simulink model "CryoDet12Chan"  (R2016b)
settings: Solver=ode45  StartTime=0.0  StopTime=10e-4  MaxStep=1e-9  RelTol=1e-3
values from neighbouring files (symbols this model uses):
  Fclk = Fadc    (= 307200000)    [setupCryoFPGAxray.m]
  freqBusAddrBits = 4    [setupCryoFPGAxray.m]
  noise = exp(2i*pi*rand(1, noiseLen))    [setupCryoFPGAxray.m]
  noiseLen = 128    [setupCryoFPGAxray.m]
  noiseSteps = 32    [setupCryoFPGAxray.m]
  Tclk = 1/Fclk    (= 3.25520833333e-09)    [setupCryoFPGAxray.m]
undefined symbols (not defined in the file or in its folder): AXI4, Lite, notch, notch2, notch3, notch4, xlipgetpartsetting
libraries: xbsIndex_r4 x1191
(part 2 of 8)

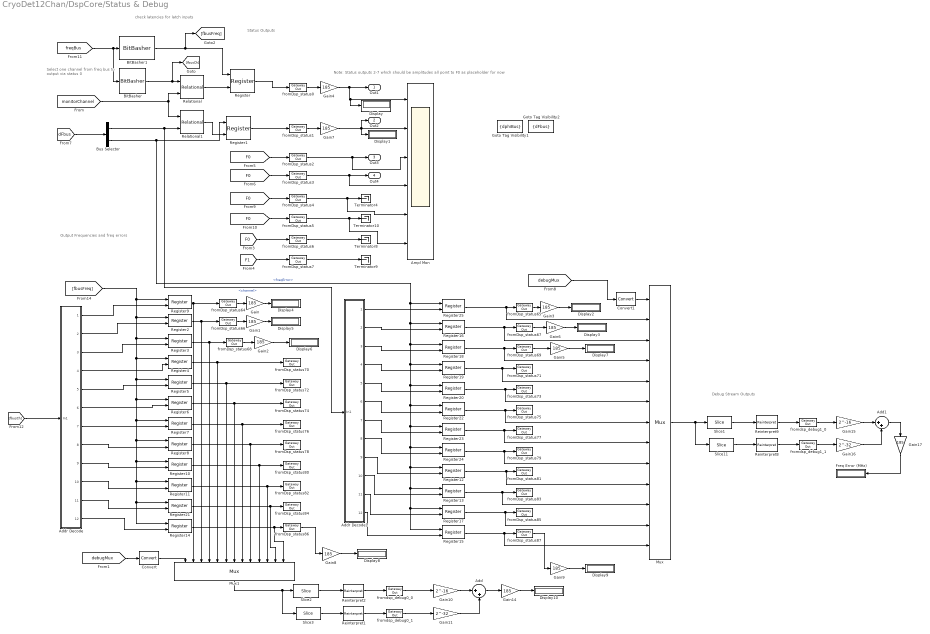
== system CryoDet12Chan/DspCore/Status & Debug ==
  note: Output Frequencies and freq errors
  note: check latencies for latch inputs
  note: Select one channel from freq bus to output via status 0
  note: Note: Status outputs 2-7 which should be amplitudes all point to F0 as placeholder for now
  note: Status Outputs
  note: Debug Stream Outputs
  Add : Sum  Inputs=|++
  Add1 : Sum  Inputs=|++
  Addr Decode : Subsystem
  Addr Decode1 : Subsystem
  Ampl Mon : Scope  NumInputPorts=6
  BitBasher : xbsIndex_r4/BitBasher  bitexpr=a={b[27:24]}  display_expr=on  sr_1=a  arith_type1=Unsigned  bin_pt1=0  sr_2=2  arith_type2=Unsigned  bin_pt2=0  sr_3=3  arith_type3=Unsigned  bin_pt3=0  sr_4=4  arith_type4=Unsigned  bin_pt4=0  dbl_ovrd=off  block_type=bitbasher
  BitBasher1 : xbsIndex_r4/BitBasher  bitexpr=a={b[23:0]}  display_expr=on  sr_1=a  arith_type1=Unsigned  bin_pt1=24  sr_2=2  arith_type2=Unsigned  bin_pt2=0  sr_3=3  arith_type3=Unsigned  bin_pt3=0  sr_4=4  arith_type4=Unsigned  bin_pt4=0  dbl_ovrd=off  block_type=bitbasher
  Bus Selector : BusSelector  OutputSignals=channel,freqError
  Convert : xbsIndex_r4/Convert  gui_display_data_type=Fixed-point  arith_type=Unsigned  n_bits=4  bin_pt=0  float_type=Single  exp_bits=8  fraction_bits=24  quantization=Truncate  overflow=Wrap  en=off  latency=1  pipeline=off  dbl_ovrd=off  block_type=convert
  Convert1 : xbsIndex_r4/Convert  gui_display_data_type=Fixed-point  arith_type=Unsigned  n_bits=4  bin_pt=0  float_type=Single  exp_bits=8  fraction_bits=24  quantization=Truncate  overflow=Wrap  en=off  latency=1  pipeline=off  dbl_ovrd=off  block_type=convert
  Display{,1..10} (11 alike) : Display
      settings: Decimation=144
  Freq Error (MHz) : Display
      settings: Decimation=144
  Gain{,1..9,14,17} (12 alike) : Gain  Gain=185
  Gain10 : Gain  Gain=2^-16
  Gain11 : Gain  Gain=2^-32
  Gain15 : Gain  Gain=2^-16
  Gain16 : Gain  Gain=2^-32
  Goto Tag Visibility1 : GotoTagVisibility  GotoTag=dphiBus
  Goto Tag Visibility2 : GotoTagVisibility  GotoTag=dFbus
  Mux : xbsIndex_r4/Mux  inputs=12  en=off  latency=0  precision=Full  arith_type=Unsigned  n_bits=16  bin_pt=14  quantization=Truncate  overflow=Wrap  dbl_ovrd=off  block_type=mux
  Mux1 : xbsIndex_r4/Mux  inputs=12  en=off  latency=0  precision=Full  arith_type=Unsigned  n_bits=16  bin_pt=14  quantization=Truncate  overflow=Wrap  dbl_ovrd=off  block_type=mux
  Register{,1..25} (26 alike) : xbsIndex_r4/Register  init=0  rst=off  en=on  dbl_ovrd=off  block_type=register
  Reinterpret{1..2,8..9} (4 alike) : xbsIndex_r4/Reinterpret  force_arith_type=on  arith_type=Unsigned  force_bin_pt=off  bin_pt=15  block_type=reinterpret
  Relational : xbsIndex_r4/Relational  mode=a=b  op_type=Bool  en=off  latency=0  dbl_ovrd=off  block_type=relational
  Relational1 : xbsIndex_r4/Relational  mode=a=b  op_type=Bool  en=off  latency=0  dbl_ovrd=off  block_type=relational
  Slice1 : xbsIndex_r4/Slice  nbits=16  boolean_output=off  mode=Upper Bit Location + Width  bit1=0  base1=MSB of Input  bit0=0  base0=LSB of Input  dbl_ovrd=off  block_type=slice
  Slice11 : xbsIndex_r4/Slice  nbits=16  boolean_output=off  mode=Lower Bit Location + Width  bit1=0  base1=MSB of Input  bit0=0  base0=LSB of Input  dbl_ovrd=off  block_type=slice
  Slice2 : xbsIndex_r4/Slice  nbits=16  boolean_output=off  mode=Upper Bit Location + Width  bit1=0  base1=MSB of Input  bit0=0  base0=LSB of Input  dbl_ovrd=off  block_type=slice
  Slice3 : xbsIndex_r4/Slice  nbits=16  boolean_output=off  mode=Lower Bit Location + Width  bit1=0  base1=MSB of Input  bit0=0  base0=LSB of Input  dbl_ovrd=off  block_type=slice
  Terminator{4,8..10} (4 alike) : Terminator
  fromDsp_status0 : xbsIndex_r4/Gateway Out  inherit_from_input=on  hdl_port=on  rows=1  columns=1  UseAsDAC=off  DACChannel='1'  interface=AXI4-Lite  automatic_assignment=off  address_offset=hex2dec('00')  intf_name=''  intf_description=''  timing_constraint=None  locs_specified=off  LOCs={}  io_standard={}  block_type=gatewayout
  fromDsp_status1 : xbsIndex_r4/Gateway Out  inherit_from_input=on  hdl_port=on  rows=1  columns=1  UseAsDAC=off  DACChannel='1'  interface=AXI4-Lite  automatic_assignment=off  address_offset=hex2dec('04')  intf_name=''  intf_description=''  timing_constraint=None  locs_specified=off  LOCs={}  io_standard={}  block_type=gatewayout
  fromDsp_status2 : xbsIndex_r4/Gateway Out  inherit_from_input=on  hdl_port=on  rows=1  columns=1  UseAsDAC=off  DACChannel='1'  interface=AXI4-Lite  automatic_assignment=off  address_offset=hex2dec('08')  intf_name=''  intf_description=''  timing_constraint=None  locs_specified=off  LOCs={}  io_standard={}  block_type=gatewayout
  fromDsp_status3 : xbsIndex_r4/Gateway Out  inherit_from_input=on  hdl_port=on  rows=1  columns=1  UseAsDAC=off  DACChannel='1'  interface=AXI4-Lite  automatic_assignment=off  address_offset=hex2dec('0C')  intf_name=''  intf_description=''  timing_constraint=None  locs_specified=off  LOCs={}  io_standard={}  block_type=gatewayout
  fromDsp_status4 : xbsIndex_r4/Gateway Out  inherit_from_input=on  hdl_port=on  rows=1  columns=1  UseAsDAC=off  DACChannel='1'  interface=AXI4-Lite  automatic_assignment=off  address_offset=hex2dec('10')  intf_name=''  intf_description=''  timing_constraint=None  locs_specified=off  LOCs={}  io_standard={}  block_type=gatewayout
  fromDsp_status5 : xbsIndex_r4/Gateway Out  inherit_from_input=on  hdl_port=on  rows=1  columns=1  UseAsDAC=off  DACChannel='1'  interface=AXI4-Lite  automatic_assignment=off  address_offset=hex2dec('14')  intf_name=''  intf_description=''  timing_constraint=None  locs_specified=off  LOCs={}  io_standard={}  block_type=gatewayout
  fromDsp_status6 : xbsIndex_r4/Gateway Out  inherit_from_input=on  hdl_port=on  rows=1  columns=1  UseAsDAC=off  DACChannel='1'  interface=AXI4-Lite  automatic_assignment=off  address_offset=hex2dec('18')  intf_name=''  intf_description=''  timing_constraint=None  locs_specified=off  LOCs={}  io_standard={}  block_type=gatewayout
  fromDsp_status64 : xbsIndex_r4/Gateway Out  inherit_from_input=on  hdl_port=on  rows=1  columns=1  UseAsDAC=off  DACChannel='1'  interface=AXI4-Lite  automatic_assignment=off  address_offset=hex2dec('100')  intf_name=''  intf_description=''  timing_constraint=None  locs_specified=off  LOCs={}  io_standard={}  block_type=gatewayout
  fromDsp_status65 : xbsIndex_r4/Gateway Out  inherit_from_input=on  hdl_port=on  rows=1  columns=1  UseAsDAC=off  DACChannel='1'  interface=AXI4-Lite  automatic_assignment=off  address_offset=hex2dec('104')  intf_name=''  intf_description=''  timing_constraint=None  locs_specified=off  LOCs={}  io_standard={}  block_type=gatewayout
  fromDsp_status66 : xbsIndex_r4/Gateway Out  inherit_from_input=on  hdl_port=on  rows=1  columns=1  UseAsDAC=off  DACChannel='1'  interface=AXI4-Lite  automatic_assignment=off  address_offset=hex2dec('108')  intf_name=''  intf_description=''  timing_constraint=None  locs_specified=off  LOCs={}  io_standard={}  block_type=gatewayout
  fromDsp_status67 : xbsIndex_r4/Gateway Out  inherit_from_input=on  hdl_port=on  rows=1  columns=1  UseAsDAC=off  DACChannel='1'  interface=AXI4-Lite  automatic_assignment=off  address_offset=hex2dec('10C')  intf_name=''  intf_description=''  timing_constraint=None  locs_specified=off  LOCs={}  io_standard={}  block_type=gatewayout
  fromDsp_status68 : xbsIndex_r4/Gateway Out  inherit_from_input=on  hdl_port=on  rows=1  columns=1  UseAsDAC=off  DACChannel='1'  interface=AXI4-Lite  automatic_assignment=off  address_offset=hex2dec('110')  intf_name=''  intf_description=''  timing_constraint=None  locs_specified=off  LOCs={}  io_standard={}  block_type=gatewayout
  fromDsp_status69 : xbsIndex_r4/Gateway Out  inherit_from_input=on  hdl_port=on  rows=1  columns=1  UseAsDAC=off  DACChannel='1'  interface=AXI4-Lite  automatic_assignment=off  address_offset=hex2dec('114')  intf_name=''  intf_description=''  timing_constraint=None  locs_specified=off  LOCs={}  io_standard={}  block_type=gatewayout
  fromDsp_status7 : xbsIndex_r4/Gateway Out  inherit_from_input=on  hdl_port=on  rows=1  columns=1  UseAsDAC=off  DACChannel='1'  interface=AXI4-Lite  automatic_assignment=off  address_offset=hex2dec('1C')  intf_name=''  intf_description=''  timing_constraint=None  locs_specified=off  LOCs={}  io_standard={}  block_type=gatewayout
  fromDsp_status70 : xbsIndex_r4/Gateway Out  inherit_from_input=on  hdl_port=on  rows=1  columns=1  UseAsDAC=off  DACChannel='1'  interface=AXI4-Lite  automatic_assignment=off  address_offset=hex2dec('118')  intf_name=''  intf_description=''  timing_constraint=None  locs_specified=off  LOCs={}  io_standard={}  block_type=gatewayout
  fromDsp_status71 : xbsIndex_r4/Gateway Out  inherit_from_input=on  hdl_port=on  rows=1  columns=1  UseAsDAC=off  DACChannel='1'  interface=AXI4-Lite  automatic_assignment=off  address_offset=hex2dec('11C')  intf_name=''  intf_description=''  timing_constraint=None  locs_specified=off  LOCs={}  io_standard={}  block_type=gatewayout
  fromDsp_status72 : xbsIndex_r4/Gateway Out  inherit_from_input=on  hdl_port=on  rows=1  columns=1  UseAsDAC=off  DACChannel='1'  interface=AXI4-Lite  automatic_assignment=off  address_offset=hex2dec('120')  intf_name=''  intf_description=''  timing_constraint=None  locs_specified=off  LOCs={}  io_standard={}  block_type=gatewayout
  fromDsp_status73 : xbsIndex_r4/Gateway Out  inherit_from_input=on  hdl_port=on  rows=1  columns=1  UseAsDAC=off  DACChannel='1'  interface=AXI4-Lite  automatic_assignment=off  address_offset=hex2dec('124')  intf_name=''  intf_description=''  timing_constraint=None  locs_specified=off  LOCs={}  io_standard={}  block_type=gatewayout
  fromDsp_status74 : xbsIndex_r4/Gateway Out  inherit_from_input=on  hdl_port=on  rows=1  columns=1  UseAsDAC=off  DACChannel='1'  interface=AXI4-Lite  automatic_assignment=off  address_offset=hex2dec('128')  intf_name=''  intf_description=''  timing_constraint=None  locs_specified=off  LOCs={}  io_standard={}  block_type=gatewayout
  fromDsp_status75 : xbsIndex_r4/Gateway Out  inherit_from_input=on  hdl_port=on  rows=1  columns=1  UseAsDAC=off  DACChannel='1'  interface=AXI4-Lite  automatic_assignment=off  address_offset=hex2dec('12C')  intf_name=''  intf_description=''  timing_constraint=None  locs_specified=off  LOCs={}  io_standard={}  block_type=gatewayout
  fromDsp_status76 : xbsIndex_r4/Gateway Out  inherit_from_input=on  hdl_port=on  rows=1  columns=1  UseAsDAC=off  DACChannel='1'  interface=AXI4-Lite  automatic_assignment=off  address_offset=hex2dec('130')  intf_name=''  intf_description=''  timing_constraint=None  locs_specified=off  LOCs={}  io_standard={}  block_type=gatewayout
  fromDsp_status77 : xbsIndex_r4/Gateway Out  inherit_from_input=on  hdl_port=on  rows=1  columns=1  UseAsDAC=off  DACChannel='1'  interface=AXI4-Lite  automatic_assignment=off  address_offset=hex2dec('134')  intf_name=''  intf_description=''  timing_constraint=None  locs_specified=off  LOCs={}  io_standard={}  block_type=gatewayout
  fromDsp_status78 : xbsIndex_r4/Gateway Out  inherit_from_input=on  hdl_port=on  rows=1  columns=1  UseAsDAC=off  DACChannel='1'  interface=AXI4-Lite  automatic_assignment=off  address_offset=hex2dec('138')  intf_name=''  intf_description=''  timing_constraint=None  locs_specified=off  LOCs={}  io_standard={}  block_type=gatewayout
  fromDsp_status79 : xbsIndex_r4/Gateway Out  inherit_from_input=on  hdl_port=on  rows=1  columns=1  UseAsDAC=off  DACChannel='1'  interface=AXI4-Lite  automatic_assignment=off  address_offset=hex2dec('13C')  intf_name=''  intf_description=''  timing_constraint=None  locs_specified=off  LOCs={}  io_standard={}  block_type=gatewayout
  fromDsp_status80 : xbsIndex_r4/Gateway Out  inherit_from_input=on  hdl_port=on  rows=1  columns=1  UseAsDAC=off  DACChannel='1'  interface=AXI4-Lite  automatic_assignment=off  address_offset=hex2dec('140')  intf_name=''  intf_description=''  timing_constraint=None  locs_specified=off  LOCs={}  io_standard={}  block_type=gatewayout
  fromDsp_status81 : xbsIndex_r4/Gateway Out  inherit_from_input=on  hdl_port=on  rows=1  columns=1  UseAsDAC=off  DACChannel='1'  interface=AXI4-Lite  automatic_assignment=off  address_offset=hex2dec('144')  intf_name=''  intf_description=''  timing_constraint=None  locs_specified=off  LOCs={}  io_standard={}  block_type=gatewayout
  fromDsp_status82 : xbsIndex_r4/Gateway Out  inherit_from_input=on  hdl_port=on  rows=1  columns=1  UseAsDAC=off  DACChannel='1'  interface=AXI4-Lite  automatic_assignment=off  address_offset=hex2dec('148')  intf_name=''  intf_description=''  timing_constraint=None  locs_specified=off  LOCs={}  io_standard={}  block_type=gatewayout
  fromDsp_status83 : xbsIndex_r4/Gateway Out  inherit_from_input=on  hdl_port=on  rows=1  columns=1  UseAsDAC=off  DACChannel='1'  interface=AXI4-Lite  automatic_assignment=off  address_offset=hex2dec('14C')  intf_name=''  intf_description=''  timing_constraint=None  locs_specified=off  LOCs={}  io_standard={}  block_type=gatewayout
  fromDsp_status84 : xbsIndex_r4/Gateway Out  inherit_from_input=on  hdl_port=on  rows=1  columns=1  UseAsDAC=off  DACChannel='1'  interface=AXI4-Lite  automatic_assignment=off  address_offset=hex2dec('150')  intf_name=''  intf_description=''  timing_constraint=None  locs_specified=off  LOCs={}  io_standard={}  block_type=gatewayout
  fromDsp_status85 : xbsIndex_r4/Gateway Out  inherit_from_input=on  hdl_port=on  rows=1  columns=1  UseAsDAC=off  DACChannel='1'  interface=AXI4-Lite  automatic_assignment=off  address_offset=hex2dec('154')  intf_name=''  intf_description=''  timing_constraint=None  locs_specified=off  LOCs={}  io_standard={}  block_type=gatewayout
  fromDsp_status86 : xbsIndex_r4/Gateway Out  inherit_from_input=on  hdl_port=on  rows=1  columns=1  UseAsDAC=off  DACChannel='1'  interface=AXI4-Lite  automatic_assignment=off  address_offset=hex2dec('158')  intf_name=''  intf_description=''  timing_constraint=None  locs_specified=off  LOCs={}  io_standard={}  block_type=gatewayout
  fromDsp_status87 : xbsIndex_r4/Gateway Out  inherit_from_input=on  hdl_port=on  rows=1  columns=1  UseAsDAC=off  DACChannel='1'  interface=AXI4-Lite  automatic_assignment=off  address_offset=hex2dec('15C')  intf_name=''  intf_description=''  timing_constraint=None  locs_specified=off  LOCs={}  io_standard={}  block_type=gatewayout
  fromdsp_debug0_0 : xbsIndex_r4/Gateway Out  inherit_from_input=on  hdl_port=on  rows=1  columns=1  UseAsDAC=off  DACChannel='1'  interface=None  automatic_assignment=on  address_offset=hex2dec('00')  intf_name=''  intf_description=''  timing_constraint=None  locs_specified=off  LOCs={}  io_standard={}  block_type=gatewayout
  fromdsp_debug0_1 : xbsIndex_r4/Gateway Out  inherit_from_input=on  hdl_port=on  rows=1  columns=1  UseAsDAC=off  DACChannel='1'  interface=None  automatic_assignment=on  address_offset=hex2dec('00')  intf_name=''  intf_description=''  timing_constraint=None  locs_specified=off  LOCs={}  io_standard={}  block_type=gatewayout
  fromdsp_debug1_0 : xbsIndex_r4/Gateway Out  inherit_from_input=on  hdl_port=on  rows=1  columns=1  UseAsDAC=off  DACChannel='1'  interface=None  automatic_assignment=on  address_offset=hex2dec('00')  intf_name=''  intf_description=''  timing_constraint=None  locs_specified=off  LOCs={}  io_standard={}  block_type=gatewayout
  fromdsp_debug1_1 : xbsIndex_r4/Gateway Out  inherit_from_input=off  hdl_port=on  rows=1  columns=1  UseAsDAC=off  DACChannel='1'  interface=None  automatic_assignment=on  address_offset=hex2dec('00')  intf_name=''  intf_description=''  timing_constraint=None  locs_specified=off  LOCs={}  io_standard={}  block_type=gatewayout
  Out1 : Outport
  Out2 : Outport  Port=2
  Out3 : Outport  Port=3
  Out4 : Outport  Port=4
  wires:
  fromDsp_status0/1 -> Gain4/1
  fromDsp_status1/1 -> Gain7/1
  fromDsp_status2/1 -> Out3/1, Ampl Mon/3
  fromDsp_status3/1 -> Out4/1, Ampl Mon/4
  fromDsp_status7/1 -> Terminator9/1
  fromDsp_status6/1 -> Terminator8/1
  [F0] -> fromDsp_status6/1
  fromDsp_status5/1 -> Ampl Mon/6, Terminator10/1
  [F1] -> fromDsp_status7/1
  [F0] -> fromDsp_status4/1
  Register1/1 -> fromDsp_status1/1
  [F0] -> fromDsp_status3/1
  [F0] -> fromDsp_status2/1
  fromDsp_status4/1 -> Ampl Mon/5, Terminator4/1
  [F0] -> fromDsp_status5/1
  fromdsp_debug0_1/1 -> Gain11/1
  fromdsp_debug0_0/1 -> Gain10/1
  Slice11/1 -> Reinterpret8/1
  Reinterpret9/1 -> fromdsp_debug1_0/1
  Slice1/1 -> Reinterpret9/1
  Reinterpret8/1 -> fromdsp_debug1_1/1
  Mux/1 -> Slice1/1, Slice11/1
  [freqBus] -> BitBasher/1, BitBasher1/1
  [monitorChannel] -> Relational1/1, Relational/2
  Relational/1 -> Register/2
  BitBasher1/1 -> [fbusFreq], Register/1
  BitBasher/1 -> [fbusCh], Relational/1
  Register/1 -> fromDsp_status0/1
  [dFbus] -> Bus Selector/1
  Bus Selector/1 -> Addr Decode1/1(In1), Relational1/2  "<channel>"
  Bus Selector/2 -> Register25/1, Register15/1, Register17/1, Register13/1, Register12/1, Register24/1, Register23/1, Register22/1, Register20/1, Register19/1, Register18/1, Register16/1, Register1/1  "<freqError>"
  Relational1/1 -> Register1/2
  Register25/1 -> Mux/2, fromDsp_status65/1
  Register16/1 -> Mux/3, fromDsp_status67/1
  Register18/1 -> Mux/4, fromDsp_status69/1
  Register19/1 -> fromDsp_status71/1, Mux/5
  Register20/1 -> Mux/6, fromDsp_status73/1
  Register22/1 -> Mux/7, fromDsp_status75/1
  Register23/1 -> Mux/8, fromDsp_status77/1
  Register24/1 -> Mux/9, fromDsp_status79/1
  Register12/1 -> Mux/10, fromDsp_status81/1
  Register13/1 -> fromDsp_status83/1, Mux/11
  Register17/1 -> Mux/12, fromDsp_status85/1
  Register15/1 -> Mux/13, fromDsp_status87/1
  [fbusCh] -> Addr Decode/1(In1)
  Addr Decode/1(Out1) -> Register9/2
  Addr Decode/2(Out2) -> Register2/2
  Addr Decode/3(Out3) -> Register3/2
  Addr Decode/4(Out4) -> Register4/2
  Addr Decode/5(Out5) -> Register5/2
  Addr Decode/6(Out6) -> Register6/2
  Addr Decode/7(Out7) -> Register7/2
  Addr Decode/8(Out8) -> Register8/2
  Addr Decode/9(Out9) -> Register10/2
  Addr Decode/10(Out10) -> Register11/2
  Addr Decode/11(Out11) -> Register21/2
  Addr Decode/12(Out12) -> Register14/2
  Register14/1 -> fromDsp_status86/1, Mux1/13
  Register21/1 -> fromDsp_status84/1, Mux1/12
  Register11/1 -> Mux1/11, fromDsp_status82/1
  Register10/1 -> Mux1/10, fromDsp_status80/1
  Register8/1 -> Mux1/9, fromDsp_status78/1
  Register7/1 -> Mux1/8, fromDsp_status76/1
  Register6/1 -> Mux1/7, fromDsp_status74/1
  Register5/1 -> Mux1/6, fromDsp_status72/1
  Register4/1 -> Mux1/5, fromDsp_status70/1
  Register3/1 -> Mux1/4, fromDsp_status68/1
  Register2/1 -> Mux1/3, fromDsp_status66/1
  [fbusFreq] -> Register9/1, Register2/1, Register4/1, Register5/1, Register6/1, Register7/1, Register8/1, Register10/1, Register11/1, Register21/1, Register14/1, Register3/1
  Addr Decode1/1(Out1) -> Register25/2
  Addr Decode1/2(Out2) -> Register16/2
  Addr Decode1/3(Out3) -> Register18/2
  Addr Decode1/4(Out4) -> Register19/2
  Addr Decode1/5(Out5) -> Register20/2
  Addr Decode1/6(Out6) -> Register22/2
  Addr Decode1/7(Out7) -> Register23/2
  Addr Decode1/8(Out8) -> Register24/2
  Addr Decode1/9(Out9) -> Register12/2
  Addr Decode1/10(Out10) -> Register13/2
  Addr Decode1/11(Out11) -> Register17/2
  Addr Decode1/12(Out12) -> Register15/2
  [debugMux] -> Convert1/1
  [debugMux] -> Convert/1
  Register9/1 -> fromDsp_status64/1, Mux1/2
  Slice3/1 -> Reinterpret1/1
  Reinterpret2/1 -> fromdsp_debug0_0/1
  Slice2/1 -> Reinterpret2/1
  Reinterpret1/1 -> fromdsp_debug0_1/1
  Mux1/1 -> Slice2/1, Slice3/1
  Convert1/1 -> Mux/1
  Convert/1 -> Mux1/1
  fromDsp_status65/1 -> Gain3/1
  fromDsp_status67/1 -> Gain6/1
  fromDsp_status64/1 -> Gain/1
  fromDsp_status66/1 -> Gain1/1
  Gain/1 -> Display4/1
  Gain1/1 -> Display5/1
  fromDsp_status68/1 -> Gain2/1
  Gain2/1 -> Display6/1
  Gain3/1 -> Display2/1
  Gain6/1 -> Display3/1
  fromDsp_status69/1 -> Gain5/1
  Gain5/1 -> Display7/1
  Gain4/1 -> Out1/1, Display/1, Ampl Mon/1
  Gain7/1 -> Display1/1, Out2/1, Ampl Mon/2
  Gain8/1 -> Display8/1
  fromDsp_status86/1 -> Gain8/1
  Gain9/1 -> Display9/1
  fromDsp_status87/1 -> Gain9/1
  Gain14/1 -> Display10/1
  Gain10/1 -> Add/1
  Add/1 -> Gain14/1
  Gain11/1 -> Add/2
  fromdsp_debug1_1/1 -> Gain16/1
  fromdsp_debug1_0/1 -> Gain15/1
  Gain17/1 -> Freq Error (MHz)/1
  Gain15/1 -> Add1/1
  Add1/1 -> Gain17/1
  Gain16/1 -> Add1/2

== system CryoDet12Chan/DspCore/AdcDac 0/Ref Delay ==
  note: Delays DAC output data used as Reference for input signal
      | Delay is to compensate for delay of DAC (big), up/downconverter, cable plant, cryostat etc.
      | This is to prevent too much delay mismatch from winding up phase vs. frequency of S21's of sidebands wrt to central line
  In1 : Inport
  Addressable Shift Register : xbsIndex_r4/Addressable Shift Register  infer_latency=on  depth=2  initVector=[0]  en=off  use_behavioral_HDL=on  Optimization=Resource  dbl_ovrd=off  block_type=addrsr
      settings: infoedit="Delay of configurable length.  Any element in the delay line can be addressed and driven onto the output port.<br><br>Hardware notes: Generates fast, compact FIFO-style shift registers or delay lines using SRL16/SRL32 mode of the slice LUTs"
  Addressable Shift Register1 : xbsIndex_r4/Addressable Shift Register  infer_latency=on  depth=2  initVector=[0]  en=off  use_behavioral_HDL=on  Optimization=Resource  dbl_ovrd=off  block_type=addrsr
      settings: infoedit="Delay of configurable length.  Any element in the delay line can be addressed and driven onto the output port.<br><br>Hardware notes: Generates fast, compact FIFO-style shift registers or delay lines using SRL16/SRL32 mode of the slice LUTs"
  Demux : Demux  Outputs=2
  Display : Display
      settings: Decimation=128
  Gateway Out : xbsIndex_r4/Gateway Out  inherit_from_input=off  hdl_port=off  rows=1  columns=1  UseAsDAC=off  DACChannel='1'  interface=None  automatic_assignment=on  address_offset=hex2dec('00')  intf_name=''  intf_description=''  timing_constraint=None  locs_specified=off  LOCs={}  io_standard={}  block_type=gatewayout
  Mux : Mux  Inputs=2
  Out1 : Outport
  wires:
  Addressable Shift Register/1 -> Mux/1
  Addressable Shift Register1/1 -> Mux/2
  In1/1 -> Demux/1
  Demux/2 -> Addressable Shift Register1/1
  Demux/1 -> Addressable Shift Register/1
  [refDel] -> Addressable Shift Register1/2, Addressable Shift Register/2, Gateway Out/1
  Mux/1 -> Out1/1
  Gateway Out/1 -> Display/1

== system CryoDet12Chan/DspCore/AdcDac 0/SBmodulator ==
  note: To DAC
  note: From tone generators
  note: to sideband demodulators
  note: Band-limited white noise
      | modulator
  note: AM generator
  note: Sideband Modulator
      | Produce sidebands at offset frequency specified by dFsb via amplitude modulation
      | Ampl1 is ratio of sidebands to central line, must be <<1
      | Also provides enable/disable for RF
      | and whitenoise modulator
  In1 : Inport
  AddSub : xbsIndex_r4/AddSub  mode=Addition  use_carryin=off  use_carryout=off  en=off  latency=1  precision=User Defined  arith_type="Signed  (2's comp)"  n_bits=16  bin_pt=15  quantization=Truncate  overflow=Wrap  use_behavioral_HDL=off  hw_selection=Fabric  pipelined=off  dbl_ovrd=off  block_type=addsub
  AddSub1 : xbsIndex_r4/AddSub  mode=Subtraction  use_carryin=off  use_carryout=off  en=off  latency=1  precision=User Defined  arith_type="Signed  (2's comp)"  n_bits=16  bin_pt=15  quantization=Truncate  overflow=Wrap  use_behavioral_HDL=off  hw_selection=Fabric  pipelined=off  dbl_ovrd=off  block_type=addsub
  Concat1 : xbsIndex_r4/Concat  num_inputs=2  dbl_ovrd=off  block_type=concat
  Constant : xbsIndex_r4/Constant  const=1.0  gui_display_data_type=Boolean  arith_type=Boolean  n_bits=16  bin_pt=14  preci_type=Single  exp_width=8  frac_width=24  explicit_period=off  period=1  equ=P=C  opselect=C  inp2=PCIN>>17  opr=+  inp1=P  carry=CIN  dbl_ovrd=off  block_type=constant
  Constant1 : xbsIndex_r4/Constant  const=1.0  gui_display_data_type=Fixed-point  arith_type=Signed (2's comp)  n_bits=16  bin_pt=15  preci_type=Single  exp_width=8  frac_width=24  explicit_period=off  period=1  equ=P=C  opselect=C  inp2=PCIN>>17  opr=+  inp1=P  carry=CIN  dbl_ovrd=off  block_type=constant
  Constant2 : xbsIndex_r4/Constant  const=0  gui_display_data_type=Fixed-point  arith_type=Signed (2's comp)  n_bits=16  bin_pt=15  preci_type=Single  exp_width=8  frac_width=24  explicit_period=off  period=1  equ=P=C  opselect=C  inp2=PCIN>>17  opr=+  inp1=P  carry=CIN  dbl_ovrd=off  block_type=constant
  Counter : xbsIndex_r4/Counter  cnt_type=Free Running  cnt_to=Inf  operation=Up  start_count=0  cnt_by_val=1  arith_type=Unsigned  n_bits=ceil(log2(noiseLen))  bin_pt=0  load_pin=off  rst=off  en=off  explicit_period=on  period=Tclk*noiseSteps  use_behavioral_HDL=off  implementation=Fabric  dbl_ovrd=off  block_type=counter
  "DDS Compiler 6.0 " : xbsIndex_r4/DDS Compiler 6.0   partspresent=Phase_Generator_and_SIN_COS_LUT  dds_clock_rate=Fclk/1e6  channels=1  mode_of_operation=Standard  modulus=9  parameter_entry=Hardware_Parameters  spurious_free_dynamic_range=45  frequency_resolution=0.4  noise_shaping=None  phase_width=16  output_width=16  output_selection=Sine_and_Cosine  negative_sine=off  negative_cosine=off  amplitude_mode=Unit_Circle  memory_type=Auto  optimization_goal=Speed  dsp48_use=Maximal  resync=off  latency_configuration=Auto  latency=5  has_phase_out=off  has_aclken=off  has_aresetn=off  explicit_period=on  period=Tclk  data_has_tlast=Not_Required  has_tready=off  s_phase_has_tuser=Not_Required  m_data_has_tuser=Not_Required  m_phase_has_tuser=Not_Required  s_phase_tuser_width=1  output_form=Twos_Complement  s_config_sync_mode=On_Vector  phase_increment=Programmable  output_frequency1=0  output_frequency2=0  output_frequency3=0  output_frequency4=0  output_frequency5=0  output_frequency6=0  output_frequency7=0  output_frequency8=0  output_frequency9=0  output_frequency10=0  output_frequency11=0  output_frequency12=0  output_frequency13=0  output_frequency14=0  output_frequency15=0  output_frequency16=0  pinc1='0'  pinc2='0'  pinc3='0'  pinc4='0'  pinc5='0'  pinc6='0'  pinc7='0'  pinc8='0'  pinc9='0'  pinc10='0'  pinc11='0'  pinc12='0'  pinc13='0'  pinc14='0'  pinc15='0'  pinc16='0'  phase_offset=None  phase_offset_angles1=0  phase_offset_angles2=0  phase_offset_angles3=0  phase_offset_angles4=0  phase_offset_angles5=0  phase_offset_angles6=0  phase_offset_angles7=0  phase_offset_angles8=0  phase_offset_angles9=0  phase_offset_angles10=0  phase_offset_angles11=0  phase_offset_angles12=0  phase_offset_angles13=0  phase_offset_angles14=0  phase_offset_angles15=0  phase_offset_angles16=0  poff1='0'  poff2='0'  poff3='0'  poff4='0'  poff5='0'  poff6='0'  poff7='0'  poff8='0'  poff9='0'  poff10='0'  poff11='0'  poff12='0'  poff13='0'  poff14='0'  poff15='0'  poff16='0'  trim_axipin_name=on  simulation_type=hybrid_sim  simulation_model=sysgen:xddsv6_0_cmodel  data_path_portlist={ 's_axis_config_tdata_poff', 's_axis_config_tdata_chan0_poff', 's_axis_config_tdata_pinc', 's_axis_config_tdata_chan0_pinc', 's_axis_phase_tdata_resync', 's_axis_phase_tdata_chan0_resync', 's_axis_phase_tdata_poff', 's_axis_phase_tdata_chan0_poff', 's_axis_phase_tdata_pinc', 's_axis_phase_tdata_chan0_pinc', 's_axis_phase_tdata_phase_in', 'm_axis_data_tdata_sine', 'm_axis_data_tdata_chan0_sine', 'm_axis_data_tdata_cosine', 'm_axis_data_tdata_chan0_cosine', 'm_axis_phase_tdata_phase_out', 'm_axis_phase_tdata_chan0_phase_out'}  por_mode=false  gui_behaviour=Sysgen  ip_name=DDS Compiler  ip_version=6.0  dsptool_ready=true  wrapper_available=true  port_translation_map={ 'aclken' => 'en', 'aresetn' => 'rst' }  ipcore_usecache=true  ipcore_useipmodelcache=true  ipcore_xco_need_fpga_part=true  ipcore_fpga_part=xlipgetpartsetting(gcb, {'kintex7', 'xc7k325t', '-3', 'fbg676'})  ipcore_verbose=false  block_type=dds_compiler_v6_0
  Demux : Demux  Outputs=2
  Gateway Out{,1..7} (8 alike) : xbsIndex_r4/Gateway Out  inherit_from_input=off  hdl_port=off  rows=1  columns=1  UseAsDAC=off  DACChannel='1'  interface=None  automatic_assignment=on  address_offset=hex2dec('00')  intf_name=''  intf_description=''  timing_constraint=None  locs_specified=off  LOCs={}  io_standard={}  block_type=gatewayout
  Modulator Control : Display
  Mult : xbsIndex_r4/Mult  precision=User Defined  arith_type="Signed  (2's comp)"  n_bits=16  bin_pt=15  quantization=Truncate  overflow=Wrap  en=off  latency=3  use_behavioral_HDL=off  opt=Speed  use_embedded=on  optimum_pipeline=off  pipeline=on  dbl_ovrd=off  use_rpm=on  placement_style=Triangular  block_type=mult
  Mult1 : xbsIndex_r4/Mult  precision=User Defined  arith_type="Signed  (2's comp)"  n_bits=16  bin_pt=15  quantization=Truncate  overflow=Wrap  en=off  latency=3  use_behavioral_HDL=off  opt=Speed  use_embedded=on  optimum_pipeline=off  pipeline=on  dbl_ovrd=off  use_rpm=on  placement_style=Triangular  block_type=mult
  Mult2 : xbsIndex_r4/Mult  precision=User Defined  arith_type="Signed  (2's comp)"  n_bits=16  bin_pt=15  quantization=Truncate  overflow=Wrap  en=off  latency=3  use_behavioral_HDL=off  opt=Speed  use_embedded=on  optimum_pipeline=off  pipeline=on  dbl_ovrd=off  use_rpm=on  placement_style=Triangular  block_type=mult
  Mux : Mux  Inputs=2
  Mux1 : xbsIndex_r4/Mux  inputs=4  en=off  latency=1  precision=User Defined  arith_type="Signed  (2's comp)"  n_bits=16  bin_pt=15  quantization=Truncate  overflow=Flag as error  dbl_ovrd=off  block_type=mux
  Mux2 : xbsIndex_r4/Mux  inputs=4  en=off  latency=1  precision=User Defined  arith_type="Signed  (2's comp)"  n_bits=16  bin_pt=15  quantization=Truncate  overflow=Flag as error  dbl_ovrd=off  block_type=mux
  Phase Modulator : Subsystem
  ROM : xbsIndex_r4/ROM  depth=noiseLen  initVector=real(noise)  distributed_mem=Block RAM  rst=off  init_reg=0  en=off  latency=1  gui_display_data_type=Fixed-point  arith_type="Signed  (2's comp)"  n_bits=16  bin_pt=15  preci_type=Single  exp_width=8  frac_width=24  optimize=Area  use_rpm=on  dbl_ovrd=off  block_type=sprom
  ROM1 : xbsIndex_r4/ROM  depth=noiseLen  initVector=imag(noise)  distributed_mem=Block RAM  rst=off  init_reg=0  en=off  latency=1  gui_display_data_type=Fixed-point  arith_type="Signed  (2's comp)"  n_bits=16  bin_pt=15  preci_type=Single  exp_width=8  frac_width=24  optimize=Area  use_rpm=on  dbl_ovrd=off  block_type=sprom
  Scope : Scope  NumInputPorts=4
  Terminator : Terminator
  sideband LO : Scope  NumInputPorts=3
  Out1 : Outport
  tag scope: SBI=global, SBQ=global
  wires:
  [dFsb] -> "DDS Compiler 6.0 "/2
  Constant/1 -> "DDS Compiler 6.0 "/1
  Mult/1 -> AddSub/1
  Constant1/1 -> AddSub1/1
  [Ampl1] -> AddSub1/2, Mult/2
  AddSub1/1 -> AddSub/2
  "DDS Compiler 6.0 "/1 -> Terminator/1
  Counter/1 -> ROM1/1, ROM/1
  Demux/1 -> Mult2/1, Phase Modulator/1(Iin)
  Demux/2 -> Phase Modulator/2(Qin), Mult1/1
  Gateway Out/1 -> Scope/1
  Gateway Out1/1 -> Scope/2
  Gateway Out2/1 -> Scope/3
  Gateway Out3/1 -> Scope/4
  "DDS Compiler 6.0 "/3 -> Gateway Out4/1, [SBI], Mult/1
  "DDS Compiler 6.0 "/2 -> Gateway Out5/1, [SBQ]
  Gateway Out4/1 -> sideband LO/1
  Gateway Out5/1 -> sideband LO/2
  [RFen] -> Concat1/2
  Concat1/1 -> Gateway Out6/1, Mux1/1, Mux2/1
  [whiteNoiseGen] -> Concat1/1
  AddSub/1 -> Gateway Out7/1, Mult1/2, Mult2/2
  ROM/1 -> Gateway Out2/1, Phase Modulator/3(Ipm)
  ROM1/1 -> Gateway Out3/1, Phase Modulator/4(Qpm)
  Constant2/1 -> Mux2/4, Mux1/2, Mux1/4, Mux2/2
  Mux2/1 -> Mux/1, Gateway Out/1
  Mux1/1 -> Mux/2, Gateway Out1/1
  Phase Modulator/1(Iout) -> Mux2/5
  Phase Modulator/2(Qout) -> Mux1/5
  Mult2/1 -> Mux2/3
  Mult1/1 -> Mux1/3
  Gateway Out6/1 -> Modulator Control/1
  Gateway Out7/1 -> sideband LO/3
  In1/1 -> Demux/1
  Mux/1 -> Out1/1

== system CryoDet12Chan/DspCore/AdcDac 0/dF ==
  note: eta Ram has latency 2
  note: sig0
  note: conj(Ref0)
  note: Match latencies
  note: dF
  note: Ref
  note: Sig
  note: Frequency error dF = Im(eta'*Ref'*Sig)
      | where eta' is like a phase and amplitude calibration including the phase determined by the 2 sidebands and amplitude determined by the reference central line and bandwidth
      |
      | get channel ID
      | fetch eta'
      | calc dF
  In1 : Inport
  etaBus : Inport  Port=2
  BW in MHz : Display
  Bus Creator : BusCreator  Inputs=2
  Bus Selector : BusSelector  OutputSignals=chanAndTvalid,signal2
  CMult : xbsIndex_r4/CMult  const=-1  gui_display_data_type=Floating-point  const_n_bits=24  const_bin_pt=22  float_type=Single  exp_bits=8  fraction_bits=24  en=off  latency=3  precision=Full  arith_type="Signed  (2's comp)"  n_bits=24  bin_pt=22  quantization=Truncate  overflow=Wrap  use_behavioral_HDL=on  mem_type=Distributed RAM  pipeline=off  dbl_ovrd=off  block_type=cmult
  Constant : xbsIndex_r4/Constant  const=0  gui_display_data_type=Fixed-point  arith_type=Unsigned  n_bits=4  bin_pt=0  preci_type=Single  exp_width=8  frac_width=24  explicit_period=off  period=1  equ=P=C  opselect=C  inp2=PCIN>>17  opr=+  inp1=P  carry=CIN  dbl_ovrd=off  block_type=constant
  Convert{,1..3,5} (5 alike) : xbsIndex_r4/Convert  gui_display_data_type=Floating-point  arith_type=Floating-point  n_bits=16  bin_pt=14  float_type=Single  exp_bits=8  fraction_bits=24  quantization=Truncate  overflow=Wrap  en=off  latency=1  pipeline=off  dbl_ovrd=off  block_type=convert
  Convert4 : xbsIndex_r4/Convert  gui_display_data_type=Fixed-point  arith_type="Signed  (2's comp)"  n_bits=32  bin_pt=30  float_type=Single  exp_bits=8  fraction_bits=24  quantization="Round  (unbiased: +/- Inf)"  overflow=Saturate  en=off  latency=1  pipeline=off  dbl_ovrd=off  block_type=convert
  CplxProd : Subsystem
  CplxProd1 : Subsystem
  Delay : xbsIndex_r4/Delay  rst=off  infoeditControl=Selection of Reset will increase slice count due to use of real FFs and instead of SRLs  en=off  latency=3  reg_retiming=on  dbl_ovrd=off  block_type=delay
  Delay1 : xbsIndex_r4/Delay  rst=off  infoeditControl=Selection of Reset will increase slice count due to use of real FFs and instead of SRLs  en=off  latency=3  reg_retiming=on  dbl_ovrd=off  block_type=delay
  Delay2 : xbsIndex_r4/Delay  rst=off  infoeditControl=Selection of Reset will increase slice count due to use of real FFs and instead of SRLs  en=off  latency=3  reg_retiming=on  dbl_ovrd=off  block_type=delay
  Delay3 : xbsIndex_r4/Delay  rst=off  infoeditControl=Selection of Reset will increase slice count due to use of real FFs and instead of SRLs  en=off  latency=20  reg_retiming=on  dbl_ovrd=off  block_type=delay
  Delay4 : xbsIndex_r4/Delay  rst=off  infoeditControl=Selection of Reset will increase slice count due to use of real FFs and instead of SRLs  en=off  latency=8  reg_retiming=on  dbl_ovrd=off  block_type=delay
  Delay5 : xbsIndex_r4/Delay  rst=off  infoeditControl=Selection of Reset will increase slice count due to use of real FFs and instead of SRLs  en=off  latency=4  reg_retiming=on  dbl_ovrd=off  block_type=delay
  Demux : Demux  Outputs=6
  Demux1 : Demux  Outputs=2
  Demux2 : Demux  Outputs=2
  Demux4 : Demux  Outputs=2
  Display2 : Display
  Display3 : Display
  Gain : Gain  Gain=185
  Gateway Out1 : xbsIndex_r4/Gateway Out  inherit_from_input=off  hdl_port=off  rows=1  columns=1  UseAsDAC=off  DACChannel='1'  interface=None  automatic_assignment=on  address_offset=hex2dec('00')  intf_name=''  intf_description=''  timing_constraint=None  locs_specified=off  LOCs={}  io_standard={}  block_type=gatewayout
  Gateway Out3 : xbsIndex_r4/Gateway Out  inherit_from_input=off  hdl_port=off  rows=1  columns=1  UseAsDAC=off  DACChannel='1'  interface=None  automatic_assignment=on  address_offset=hex2dec('00')  intf_name=''  intf_description=''  timing_constraint=None  locs_specified=off  LOCs={}  io_standard={}  block_type=gatewayout
  Gateway Out4 : xbsIndex_r4/Gateway Out  inherit_from_input=off  hdl_port=off  rows=1  columns=1  UseAsDAC=off  DACChannel='1'  interface=None  automatic_assignment=on  address_offset=hex2dec('00')  intf_name=''  intf_description=''  timing_constraint=None  locs_specified=off  LOCs={}  io_standard={}  block_type=gatewayout
  Goto Tag Visibility2 : GotoTagVisibility  GotoTag=dFbus
  Mult4 : xbsIndex_r4/Mult  precision=Full  arith_type="Signed  (2's comp)"  n_bits=32  bin_pt=30  quantization="Round  (unbiased: +/- Inf)"  overflow=Saturate  en=off  latency=3  use_behavioral_HDL=off  opt=Speed  use_embedded=on  optimum_pipeline=off  pipeline=on  dbl_ovrd=off  use_rpm=on  placement_style=Triangular  block_type=mult
  Register : xbsIndex_r4/Register  init=0  rst=off  en=on  dbl_ovrd=off  block_type=register
  Relational : xbsIndex_r4/Relational  mode=a=b  op_type=Bool  en=off  latency=0  dbl_ovrd=off  block_type=relational
  Terminator{,2,4..7} (6 alike) : Terminator
  Toolbar : xbsIndex_r4/Toolbar  func=xltoolbar  block_type=toolbar
      settings: infoedit=Toolbar
  dF output : Scope  NumInputPorts=2
  etaRAM : Subsystem
  Out1 : Outport
  tag scope: dFbus=global
  wires:
  Demux/1 -> Demux1/1
  Demux/4 -> Demux2/1
  CMult/1 -> CplxProd/4(Im_B)
  Demux2/1 -> Convert2/1
  Demux2/2 -> Convert3/1
  Delay/1 -> CplxProd/5(Re_B)
  Demux1/2 -> Convert1/1
  Demux1/1 -> Convert/1
  Delay1/1 -> CplxProd/2(Im_A)
  CplxProd1/3(Re_Out) -> Terminator/1
  CplxProd1/1(tvalidOut) -> Terminator2/1
  In1/1 -> Bus Selector/1
  Bus Creator/1 -> [dFbus], Out1/1
  Convert5/1 -> Gateway Out1/1, Mult4/1
  CplxProd1/2(Im_Out) -> Mult4/2
  Demux/3 -> Terminator5/1
  Demux/2 -> Terminator4/1
  Demux/5 -> Terminator6/1
  Demux/6 -> Terminator7/1
  Demux4/1 -> Delay3/1, Delay4/1
  Demux4/2 -> Delay5/1
  Bus Selector/1 -> Demux4/1  "<chanAndTvalid>"
  Bus Selector/2 -> Demux/1  "<signal2>"
  etaBus/1 -> etaRAM/2("etaBusIn ")
  Delay4/1 -> etaRAM/1(readAddr)
  Mult4/1 -> Convert4/1  "freqError"
  Delay3/1 -> Bus Creator/1, Relational/1, Gateway Out3/1  "channel"
  Convert3/1 -> Delay/1
  Convert2/1 -> CMult/1
  Convert1/1 -> Delay2/1
  Convert/1 -> Delay1/1
  Delay2/1 -> CplxProd/3(Re_A)
  Delay5/1 -> CplxProd/1(tvalidIn)
  CplxProd/2(Im_Out) -> CplxProd1/2(Im_A)
  CplxProd/3(Re_Out) -> CplxProd1/3(Re_A)
  etaRAM/1(etaQ) -> CplxProd1/4(Im_B)
  etaRAM/2(etaI) -> CplxProd1/5(Re_B)
  CplxProd/1(tvalidOut) -> CplxProd1/1(tvalidIn)
  Convert4/1 -> Register/1, Bus Creator/2  "freqError"
  Gateway Out4/1 -> Display3/1, dF output/2
  Gateway Out3/1 -> dF output/1, Display2/1
  Constant/1 -> Relational/2
  Relational/1 -> Register/2
  Register/1 -> Gateway Out4/1
  [BW] -> Convert5/1
  Gateway Out1/1 -> Gain/1
  Gain/1 -> BW in MHz/1

== system CryoDet12Chan/DspCore/AdcDac 0/dphi ==
  note: check format of Fbus
  note: scale by 1/2 since phase increment per 1/370 = 1/2 of phase increment per 1/185
  note: dPhi
      | calculate complex phase advance for a single sample of ADC input
      | at the frequency of a single channel and send off on dphiBus
  In1 : Inport
  BitBasher : xbsIndex_r4/BitBasher  bitexpr=a={1'b0, b[23:1]}  display_expr=on  sr_1=a  arith_type1=Unsigned  bin_pt1=24  sr_2=2  arith_type2=Unsigned  bin_pt2=0  sr_3=3  arith_type3=Unsigned  bin_pt3=0  sr_4=4  arith_type4=Unsigned  bin_pt4=0  dbl_ovrd=off  block_type=bitbasher
  Bus Creator : BusCreator  Inputs=3
  Constant : xbsIndex_r4/Constant  const=1  gui_display_data_type=Boolean  arith_type=Boolean  n_bits=16  bin_pt=14  preci_type=Single  exp_width=8  frac_width=24  explicit_period=off  period=1  equ=P=C  opselect=C  inp2=PCIN>>17  opr=+  inp1=P  carry=CIN  dbl_ovrd=off  block_type=constant
  Convert : xbsIndex_r4/Convert  gui_display_data_type=Fixed-point  arith_type=Unsigned  n_bits=16  bin_pt=16  float_type=Single  exp_bits=8  fraction_bits=24  quantization="Round  (unbiased: Even Values)"  overflow=Wrap  en=off  latency=1  pipeline=off  dbl_ovrd=off  block_type=convert
  "DDS Compiler 6.0 " : xbsIndex_r4/DDS Compiler 6.0   partspresent=SIN_COS_LUT_only  dds_clock_rate=100  channels=1  mode_of_operation=Standard  modulus=9  parameter_entry=Hardware_Parameters  spurious_free_dynamic_range=45  frequency_resolution=0.4  noise_shaping=None  phase_width=16  output_width=IQbits  output_selection=Sine_and_Cosine  negative_sine=off  negative_cosine=off  amplitude_mode=Unit_Circle  memory_type=Auto  optimization_goal=Speed  dsp48_use=Maximal  resync=off  latency_configuration=Auto  latency=15  has_phase_out=off  has_aclken=off  has_aresetn=off  explicit_period=on  period=Tclk  data_has_tlast=Not_Required  has_tready=off  s_phase_has_tuser=Not_Required  m_data_has_tuser=Not_Required  m_phase_has_tuser=Not_Required  s_phase_tuser_width=1  output_form=Twos_Complement  s_config_sync_mode=On_Vector  phase_increment=Fixed  output_frequency1=0  output_frequency2=0  output_frequency3=0  output_frequency4=0  output_frequency5=0  output_frequency6=0  output_frequency7=0  output_frequency8=0  output_frequency9=0  output_frequency10=0  output_frequency11=0  output_frequency12=0  output_frequency13=0  output_frequency14=0  output_frequency15=0  output_frequency16=0  pinc1='0'  pinc2='0'  pinc3='0'  pinc4='0'  pinc5='0'  pinc6='0'  pinc7='0'  pinc8='0'  pinc9='0'  pinc10='0'  pinc11='0'  pinc12='0'  pinc13='0'  pinc14='0'  pinc15='0'  pinc16='0'  phase_offset=Programmable  phase_offset_angles1=0  phase_offset_angles2=0  phase_offset_angles3=0  phase_offset_angles4=0  phase_offset_angles5=0  phase_offset_angles6=0  phase_offset_angles7=0  phase_offset_angles8=0  phase_offset_angles9=0  phase_offset_angles10=0  phase_offset_angles11=0  phase_offset_angles12=0  phase_offset_angles13=0  phase_offset_angles14=0  phase_offset_angles15=0  phase_offset_angles16=0  poff1='0'  poff2='0'  poff3='0'  poff4='0'  poff5='0'  poff6='0'  poff7='0'  poff8='0'  poff9='0'  poff10='0'  poff11='0'  poff12='0'  poff13='0'  poff14='0'  poff15='0'  poff16='0'  trim_axipin_name=on  simulation_type=hybrid_sim  simulation_model=sysgen:xddsv6_0_cmodel  data_path_portlist={ 's_axis_config_tdata_poff', 's_axis_config_tdata_chan0_poff', 's_axis_config_tdata_pinc', 's_axis_config_tdata_chan0_pinc', 's_axis_phase_tdata_resync', 's_axis_phase_tdata_chan0_resync', 's_axis_phase_tdata_poff', 's_axis_phase_tdata_chan0_poff', 's_axis_phase_tdata_pinc', 's_axis_phase_tdata_chan0_pinc', 's_axis_phase_tdata_phase_in', 'm_axis_data_tdata_sine', 'm_axis_data_tdata_chan0_sine', 'm_axis_data_tdata_cosine', 'm_axis_data_tdata_chan0_cosine', 'm_axis_phase_tdata_phase_out', 'm_axis_phase_tdata_chan0_phase_out'}  por_mode=false  gui_behaviour=Sysgen  ip_name=DDS Compiler  ip_version=6.0  dsptool_ready=true  wrapper_available=true  port_translation_map={ 'aclken' => 'en', 'aresetn' => 'rst' }  ipcore_usecache=true  ipcore_useipmodelcache=true  ipcore_xco_need_fpga_part=true  ipcore_fpga_part=xlipgetpartsetting(gcb, {'kintex7', 'xc7k325t', '-3', 'fbg676'})  ipcore_verbose=false  block_type=dds_compiler_v6_0
  Delay : xbsIndex_r4/Delay  rst=off  infoeditControl=Selection of Reset will increase slice count due to use of real FFs and instead of SRLs  en=off  latency=7  reg_retiming=off  dbl_ovrd=off  block_type=delay
  Display : Display
  Display1 : Display
  Display2 : Display
  Gateway Out{,1..6} (7 alike) : xbsIndex_r4/Gateway Out  inherit_from_input=off  hdl_port=off  rows=1  columns=1  UseAsDAC=off  DACChannel='1'  interface=None  automatic_assignment=on  address_offset=hex2dec('00')  intf_name=''  intf_description=''  timing_constraint=None  locs_specified=off  LOCs={}  io_standard={}  block_type=gatewayout
  Slice : xbsIndex_r4/Slice  nbits=freqBusAddrBits  boolean_output=off  mode=Lower Bit Location + Width  bit1=0  base1=MSB of Input  bit0=freqBits  base0=LSB of Input  dbl_ovrd=off  block_type=slice
  dphi scope : Scope  NumInputPorts=3
  dphi scope1 : Scope  NumInputPorts=3
  tag scope: dphiBus=scoped
  wires:
  Bus Creator/1 -> [dphiBus]
  BitBasher/1 -> Convert/1, Gateway Out4/1
  Delay/1 -> Bus Creator/1, Gateway Out6/1, Gateway Out2/1  "channel"
  Convert/1 -> Gateway Out5/1, "DDS Compiler 6.0 "/2
  Constant/1 -> "DDS Compiler 6.0 "/1
  "DDS Compiler 6.0 "/2 -> Bus Creator/2, Gateway Out/1  "dPhiQ"
  "DDS Compiler 6.0 "/3 -> Bus Creator/3, Gateway Out1/1  "dPhiI"
  Gateway Out/1 -> dphi scope/2, Display/1
  Gateway Out1/1 -> dphi scope/3, Display1/1
  Gateway Out2/1 -> Display2/1
  In1/1 -> BitBasher/1, Slice/1
  Slice/1 -> Gateway Out3/1, Delay/1
  Gateway Out5/1 -> dphi scope1/3
  Gateway Out4/1 -> dphi scope1/2
  Gateway Out3/1 -> dphi scope1/1
  Gateway Out6/1 -> dphi scope/1
